simulink model "cruiseControl"  (R2019b)
settings: Solver=VariableStepAuto  StartTime=0.0  StopTime=10.0  RelTol=1e-3
settings Model: Creator=benmacnaughton  LastModifiedBy=benmacnaughton

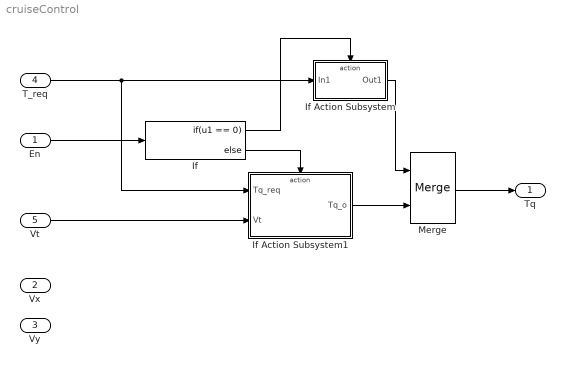
== system cruiseControl ==
  En : Inport
  Vx : Inport  Port=2
  Vy : Inport  Port=3
  T_req : Inport  Port=4
  Vt : Inport  Port=5
  If : If  IfExpression=u1 == 0
  If Action Subsystem : Subsystem  TreatAsAtomicUnit=on
  If Action Subsystem1 : Subsystem  TreatAsAtomicUnit=on
  Merge : Merge
  Tq : Outport
  wires:
  En/1 -> If/1
  T_req/1 -> If Action Subsystem1/1(Tq_req), If Action Subsystem/1(In1)
  If/1 -> If Action Subsystem/Action
  If Action Subsystem/1(Out1) -> Merge/1
  Merge/1 -> Tq/1
  Vt/1 -> If Action Subsystem1/2(Vt)
  If/2 -> If Action Subsystem1/Action
  If Action Subsystem1/1(Tq_o) -> Merge/2

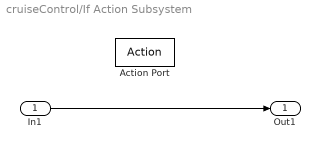
== system cruiseControl/If Action Subsystem ==
  In1 : Inport
  Action Port : ActionPort  ActionPortLabel=if(u1 == 0)
  Out1 : Outport
  wires:
  In1/1 -> Out1/1

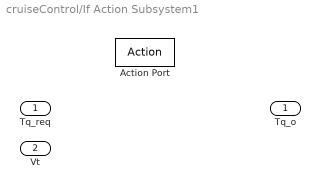
== system cruiseControl/If Action Subsystem1 ==
  Tq_req : Inport
  Vt : Inport  Port=2
  Action Port : ActionPort  ActionPortLabel=else
  Tq_o : Outport
